simulink model "bmgen_array_N20"  (R2014a)
settings: Solver=ode45  StartTime=0.0  StopTime=Tmax  RelTol=1e-3
values from neighbouring files (symbols this model uses):
  Tgrid = (1 / Fgrid)    (= 0.0166666666667)    [array_init.m]
  Ts = Tthd    (= 1.66666666667e-05)    [array_init.m]
  Tstartup = 3e-3    (= 0.003)    [array_init.m]
  Vgrid = (sqrt(2)*Vgridrms)    [array_init.m]
undefined symbols (not defined in the file or in its folder): Acarray, Adarray, Aoarray, Bcarray, Bdarray, Boarray, Carray, Darray, Larray, N, Rarray, TswitchArray
libraries: module_switch x20, powerlib_meascontrol x3
settings Model: Creator=tjohnson  LastModifiedBy=tjohnson

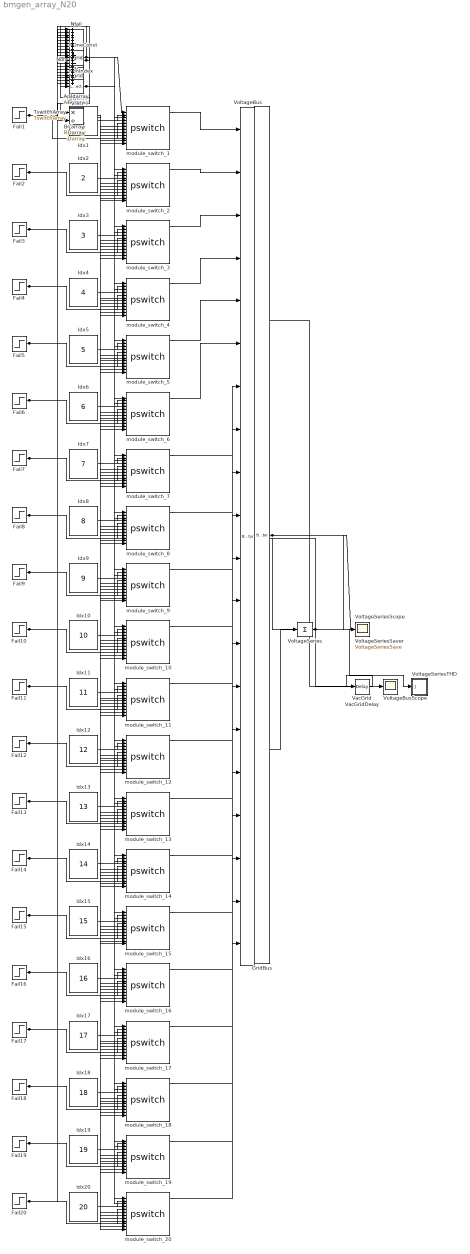
== system bmgen_array_N20 ==
  Acarray : Constant  Value=Acarray
  Adarray : Constant  Value=Adarray
  Aoarray : Constant  Value=Aoarray
  Bcarray : Constant  Value=Bcarray
  Bdarray : Constant  Value=Bdarray
  Boarray : Constant  Value=Boarray
  Carray : Constant  Value=Carray
  Darray : Constant  Value=Darray
  Fail{1..20} (20 alike) : Step  Time=0  After=0
  GridBus : BusCreator  Inputs=2
  Idx1 : Constant
  Idx10 : Constant  Value=10
  Idx11 : Constant  Value=11
  Idx12 : Constant  Value=12
  Idx13 : Constant  Value=13
  Idx14 : Constant  Value=14
  Idx15 : Constant  Value=15
  Idx16 : Constant  Value=16
  Idx17 : Constant  Value=17
  Idx18 : Constant  Value=18
  Idx19 : Constant  Value=19
  Idx2 : Constant  Value=2
  Idx20 : Constant  Value=20
  Idx3 : Constant  Value=3
  Idx4 : Constant  Value=4
  Idx5 : Constant  Value=5
  Idx6 : Constant  Value=6
  Idx7 : Constant  Value=7
  Idx8 : Constant  Value=8
  Idx9 : Constant  Value=9
  Larray : Constant  Value=Larray
  N : Constant  Value=N
  NOneConst : Constant
  Nfail : Sum  Inputs=++++++++++++++++++++  SaturateOnIntegerOverflow=on  InputSameDT=on  OutDataTypeStr=Inherit: Same as first input
  Non : Sum  Inputs=+-  SaturateOnIntegerOverflow=on  InputSameDT=on  OutDataTypeStr=Inherit: Same as first input
  NonIndex : Sum  Inputs=+-  SaturateOnIntegerOverflow=on  InputSameDT=on  OutDataTypeStr=Inherit: Same as first input
  Rarray : Constant  Value=Rarray
  TSwitch : LookupNDDirect  NumberOfTableDimensions=3  InputsSelectThisObjectFromTable=2-D Matrix  Table=TswitchArray
  TswitchArray : Constant  Value=TswitchArray
  VacGrid : Sin  Amplitude=Vgrid  Frequency=2*pi/Tgrid
  VacGridDelay : TransportDelay  DelayTime=Tstartup
  Vgrid : Constant  Value=Vgrid
  VoltageBus : BusCreator  Inputs=N
  VoltageBusScope : Scope
      settings: SaveName=ScopeDataSwitching
  VoltageSeries : Sum  Inputs=+  SaturateOnIntegerOverflow=on  InputSameDT=on  OutDataTypeStr=Inherit: Same as first input
  VoltageSeriesSaver : ToWorkspace  VariableName=VoltageSeriesSave
  VoltageSeriesScope : Scope
      settings: SaveName=ScopeDataSeries
  VoltageSeriesTHD : Subsystem  VariantControl=Variant1
  Vref : Product  Inputs=*/  SaturateOnIntegerOverflow=on  RndMeth=Zero  InputSameDT=on  OutDataTypeStr=Inherit: Same as first input
  module_switch_{1..20} (20 alike) : module_switch/pswitch
  wires:
  VacGrid/1 -> VacGridDelay/1
  VacGridDelay/1 -> GridBus/1
  N/1 -> Non/1, module_switch_1/1, module_switch_2/1, module_switch_3/1, module_switch_4/1, module_switch_5/1, module_switch_6/1, module_switch_7/1, module_switch_8/1, module_switch_9/1, module_switch_10/1, module_switch_11/1, module_switch_12/1, module_switch_13/1, module_switch_14/1, module_switch_15/1, module_switch_16/1, module_switch_17/1, module_switch_18/1, module_switch_19/1, module_switch_20/1
  Nfail/1 -> Non/2
  Non/1 -> NonIndex/1, Vref/2
  NOneConst/1 -> NonIndex/2
  Vgrid/1 -> Vref/1
  NonIndex/1 -> TSwitch/1
  VoltageSeries/1 -> GridBus/2, VoltageSeriesTHD/1(In1)
  VoltageBus/1 -> VoltageSeries/1, VoltageBusScope/1
  GridBus/1 -> VoltageSeriesScope/1, VoltageSeriesSaver/1
  Idx1/1 -> module_switch_1/2
  Fail1/1 -> module_switch_1/5, Nfail/1
  TSwitch/1 -> module_switch_1/3, module_switch_2/3, module_switch_3/3, module_switch_4/3, module_switch_5/3, module_switch_6/3, module_switch_7/3, module_switch_8/3, module_switch_9/3, module_switch_10/3, module_switch_11/3, module_switch_12/3, module_switch_13/3, module_switch_14/3, module_switch_15/3, module_switch_16/3, module_switch_17/3, module_switch_18/3, module_switch_19/3, module_switch_20/3
  Darray/1 -> module_switch_1/4, module_switch_2/4, module_switch_3/4, module_switch_4/4, module_switch_5/4, module_switch_6/4, module_switch_7/4, module_switch_8/4, module_switch_9/4, module_switch_10/4, module_switch_11/4, module_switch_12/4, module_switch_13/4, module_switch_14/4, module_switch_15/4, module_switch_16/4, module_switch_17/4, module_switch_18/4, module_switch_19/4, module_switch_20/4
  Acarray/1 -> module_switch_1/6, module_switch_2/6, module_switch_3/6, module_switch_4/6, module_switch_5/6, module_switch_6/6, module_switch_7/6, module_switch_8/6, module_switch_9/6, module_switch_10/6, module_switch_11/6, module_switch_12/6, module_switch_13/6, module_switch_14/6, module_switch_15/6, module_switch_16/6, module_switch_17/6, module_switch_18/6, module_switch_19/6, module_switch_20/6
  Aoarray/1 -> module_switch_1/7, module_switch_2/7, module_switch_3/7, module_switch_4/7, module_switch_5/7, module_switch_6/7, module_switch_7/7, module_switch_8/7, module_switch_9/7, module_switch_10/7, module_switch_11/7, module_switch_12/7, module_switch_13/7, module_switch_14/7, module_switch_15/7, module_switch_16/7, module_switch_17/7, module_switch_18/7, module_switch_19/7, module_switch_20/7
  Adarray/1 -> module_switch_1/11, module_switch_2/11, module_switch_3/11, module_switch_4/11, module_switch_5/11, module_switch_6/11, module_switch_7/11, module_switch_8/11, module_switch_9/11, module_switch_10/11, module_switch_11/11, module_switch_12/11, module_switch_13/11, module_switch_14/11, module_switch_15/11, module_switch_16/11, module_switch_17/11, module_switch_18/11, module_switch_19/11, module_switch_20/11
  Bcarray/1 -> module_switch_1/9, module_switch_2/9, module_switch_3/9, module_switch_4/9, module_switch_5/9, module_switch_6/9, module_switch_7/9, module_switch_8/9, module_switch_9/9, module_switch_10/9, module_switch_11/9, module_switch_12/9, module_switch_13/9, module_switch_14/9, module_switch_15/9, module_switch_16/9, module_switch_17/9, module_switch_18/9, module_switch_19/9, module_switch_20/9
  Boarray/1 -> module_switch_1/8, module_switch_2/8, module_switch_3/8, module_switch_4/8, module_switch_5/8, module_switch_6/8, module_switch_7/8, module_switch_8/8, module_switch_9/8, module_switch_10/8, module_switch_11/8, module_switch_12/8, module_switch_13/8, module_switch_14/8, module_switch_15/8, module_switch_16/8, module_switch_17/8, module_switch_18/8, module_switch_19/8, module_switch_20/8
  Bdarray/1 -> module_switch_1/12, module_switch_2/12, module_switch_3/12, module_switch_4/12, module_switch_5/12, module_switch_6/12, module_switch_7/12, module_switch_8/12, module_switch_9/12, module_switch_10/12, module_switch_11/12, module_switch_12/12, module_switch_13/12, module_switch_14/12, module_switch_15/12, module_switch_16/12, module_switch_17/12, module_switch_18/12, module_switch_19/12, module_switch_20/12
  Vref/1 -> module_switch_1/10, module_switch_2/10, module_switch_3/10, module_switch_4/10, module_switch_5/10, module_switch_6/10, module_switch_7/10, module_switch_8/10, module_switch_9/10, module_switch_10/10, module_switch_11/10, module_switch_12/10, module_switch_13/10, module_switch_14/10, module_switch_15/10, module_switch_16/10, module_switch_17/10, module_switch_18/10, module_switch_19/10, module_switch_20/10
  module_switch_1/1 -> VoltageBus/1
  Idx2/1 -> module_switch_2/2
  Fail2/1 -> module_switch_2/5, Nfail/2
  module_switch_2/1 -> VoltageBus/2
  Idx3/1 -> module_switch_3/2
  Fail3/1 -> module_switch_3/5, Nfail/3
  module_switch_3/1 -> VoltageBus/3
  Idx4/1 -> module_switch_4/2
  Fail4/1 -> module_switch_4/5, Nfail/4
  module_switch_4/1 -> VoltageBus/4
  Idx5/1 -> module_switch_5/2
  Fail5/1 -> module_switch_5/5, Nfail/5
  module_switch_5/1 -> VoltageBus/5
  Idx6/1 -> module_switch_6/2
  Fail6/1 -> module_switch_6/5, Nfail/6
  module_switch_6/1 -> VoltageBus/6
  Idx7/1 -> module_switch_7/2
  Fail7/1 -> module_switch_7/5, Nfail/7
  module_switch_7/1 -> VoltageBus/7
  Idx8/1 -> module_switch_8/2
  Fail8/1 -> module_switch_8/5, Nfail/8
  module_switch_8/1 -> VoltageBus/8
  Idx9/1 -> module_switch_9/2
  Fail9/1 -> module_switch_9/5, Nfail/9
  module_switch_9/1 -> VoltageBus/9
  Idx10/1 -> module_switch_10/2
  Fail10/1 -> module_switch_10/5, Nfail/10
  module_switch_10/1 -> VoltageBus/10
  Idx11/1 -> module_switch_11/2
  Fail11/1 -> module_switch_11/5, Nfail/11
  module_switch_11/1 -> VoltageBus/11
  Idx12/1 -> module_switch_12/2
  Fail12/1 -> module_switch_12/5, Nfail/12
  module_switch_12/1 -> VoltageBus/12
  Idx13/1 -> module_switch_13/2
  Fail13/1 -> module_switch_13/5, Nfail/13
  module_switch_13/1 -> VoltageBus/13
  Idx14/1 -> module_switch_14/2
  Fail14/1 -> module_switch_14/5, Nfail/14
  module_switch_14/1 -> VoltageBus/14
  Idx15/1 -> module_switch_15/2
  Fail15/1 -> module_switch_15/5, Nfail/15
  module_switch_15/1 -> VoltageBus/15
  Idx16/1 -> module_switch_16/2
  Fail16/1 -> module_switch_16/5, Nfail/16
  module_switch_16/1 -> VoltageBus/16
  Idx17/1 -> module_switch_17/2
  Fail17/1 -> module_switch_17/5, Nfail/17
  module_switch_17/1 -> VoltageBus/17
  Idx18/1 -> module_switch_18/2
  Fail18/1 -> module_switch_18/5, Nfail/18
  module_switch_18/1 -> VoltageBus/18
  Idx19/1 -> module_switch_19/2
  Fail19/1 -> module_switch_19/5, Nfail/19
  module_switch_19/1 -> VoltageBus/19
  Idx20/1 -> module_switch_20/2
  Fail20/1 -> module_switch_20/5, Nfail/20
  module_switch_20/1 -> VoltageBus/20

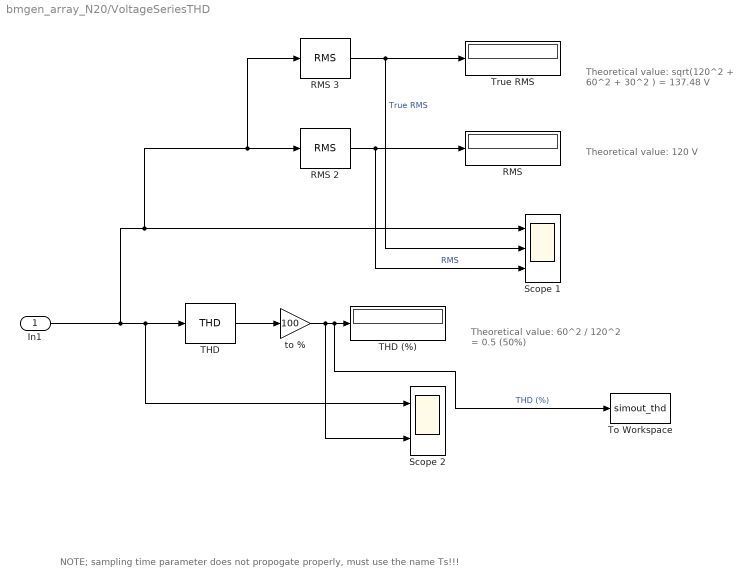
== system bmgen_array_N20/VoltageSeriesTHD ==
  note: NOTE; sampling time parameter does not propogate properly, must use the name Ts!!!
  note: Theoretical value:
      | 60^2 / 120^2 = 0.5  (50%)
  note: Theoretical value:
      | sqrt(120^2 + 60^2 + 30^2 )
      | = 137.48 V
  note: Theoretical value:
      | 120 V
  In1 : Inport
  RMS : Display
      settings: Format=bank
  RMS 2 : powerlib_meascontrol/Measurements/RMS  TrueRMS=off  Freq=Fgrid  RMSInit=Vgridrms  Ts=Ts
  RMS 3 : powerlib_meascontrol/Measurements/RMS  TrueRMS=on  Freq=Fgrid  RMSInit=Vgridrms  Ts=Ts
  Scope 1 : Scope  NumInputPorts=3
      settings: TimeRange=0.1  YMin=-250~50~50  YMax=250~150~150  SaveName=ScopeData2
  Scope 2 : Scope  NumInputPorts=2
      settings: TimeRange=0.0333333  YMin=-550~0  YMax=500~50
  THD : powerlib_meascontrol/Measurements/THD  Freq=Fgrid  Ts=Ts
  THD (%) : Display
      settings: Format=bank
  To Workspace : ToWorkspace  VariableName=simout_thd  SaveFormat=Timeseries  SampleTime=-1
  True RMS : Display
      settings: Format=bank
  to % : Gain  Gain=100  SampleTime=Ts
  wires:
  THD/1 -> to %/1
  to %/1 -> THD (%)/1, To Workspace/1, Scope 2/2  "THD (%)"
  In1/1 -> RMS 2/1, RMS 3/1, Scope 1/1, Scope 2/1, THD/1
  RMS 2/1 -> RMS/1, Scope 1/3  "RMS"
  RMS 3/1 -> True RMS/1, Scope 1/2  "True RMS"
